simulink model "flyback"  (R2022b)
settings: Solver=FixedStepAuto  StartTime=0.0  StopTime=0.1  FixedStep=1e-7  RelTol=1e-3
values from neighbouring files (symbols this model uses):
  C = Vo*d/(delta_Vc*R*fsw)    (= 0.000104166666667)    [flyback.m]
  d = d*100    (= 37.5)    [flyback.m]
  fsw = 50e3    (= 50000)    [flyback.m]
  Lm = abs(Vin*d/(delta_iL*fsw))    [flyback.m]
  n = 1/5    (= 0.2)    [flyback.m]
  R = Vo^2/Po    (= 7.2)    [flyback.m]
libraries: spsCurrentMeasurementLib x8, spsVoltageMeasurementLib x6, spsParallelRLCBranchLib x3, spsDCVoltageSourceLib x1, spsDiodeLib x1, spsIGBTLib x1, spsVariableRatioTransformerLib x1, sps_lib x1
settings Model: Creator=isild  LastModifiedBy=isild

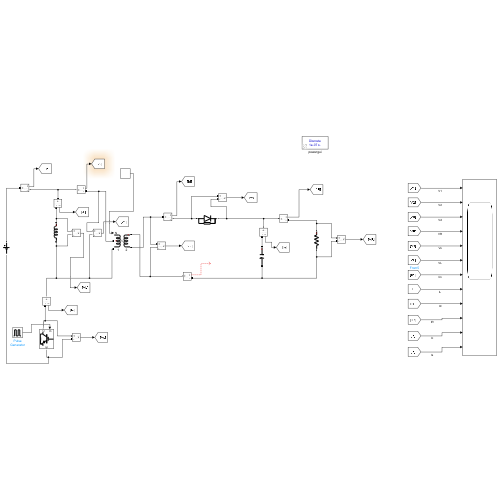
[thumbnail: Simulink's stored preview of the top-level diagram]
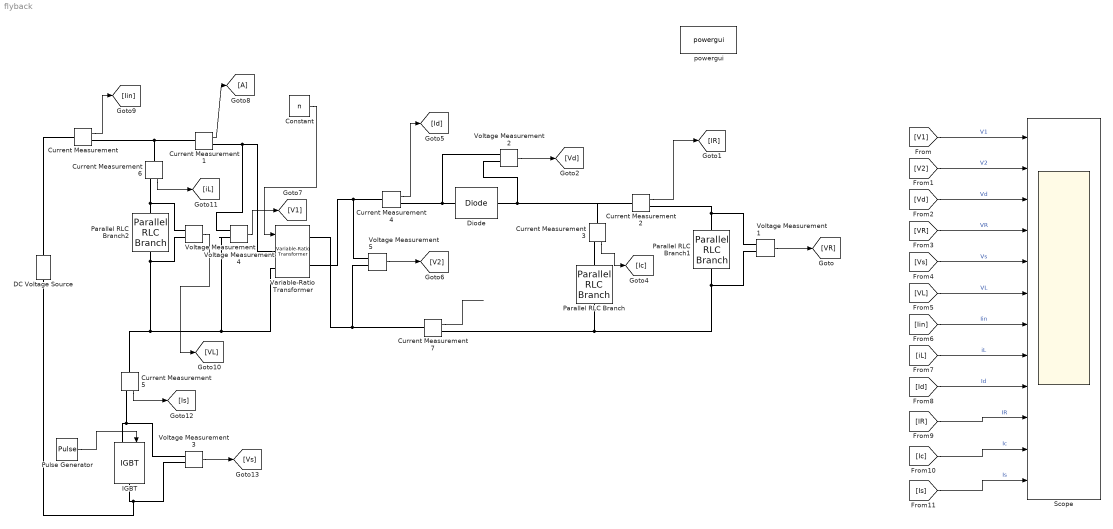
== system flyback ==
  Constant : Constant  Value=n
  Current Measurement{,1..7} (8 alike) : spsCurrentMeasurementLib/Current Measurement  PhasorSimulation=off  OutputType=Complex  PSBequivalent=0
  DC Voltage Source : spsDCVoltageSourceLib/DC Voltage Source  Amplitude=100  Measurements=None
  Diode : spsDiodeLib/Diode  Ron=0.001  Lon=0  Vf=0.8  IC=0  UseSnubber=0  Rs=500  Cs=250e-9  Measurements=off
  Goto8 : Goto
  IGBT : spsIGBTLib/IGBT  Ron=0.001  Lon=0  Vf=1  Tf=1e-6  Tt=2e-6  IC=0  Rs=1e5  Cs=inf  Measurements=off
  Parallel RLC Branch : spsParallelRLCBranchLib/Parallel RLC Branch  LConnTagsString=a  RConnTagsString=__new0  BranchType=C  Resistance=1  Inductance=1e-3  SetiL0=off  InitialCurrent=0  Capacitance=C  Setx0=off  InitialVoltage=0  Measurements=None
  Parallel RLC Branch1 : spsParallelRLCBranchLib/Parallel RLC Branch  LConnTagsString=a  RConnTagsString=__new0  BranchType=R  Resistance=R  Inductance=1e-3  SetiL0=off  InitialCurrent=0  Capacitance=1e-6  Setx0=off  InitialVoltage=0  Measurements=None
  Parallel RLC Branch2 : spsParallelRLCBranchLib/Parallel RLC Branch  LConnTagsString=a  RConnTagsString=__new0  BranchType=L  Resistance=1  Inductance=Lm  SetiL0=off  InitialCurrent=0  Capacitance=1e-6  Setx0=off  InitialVoltage=0  Measurements=None
  Pulse Generator : DiscretePulseGenerator  PulseType=Time based  Period=1/fsw  PulseWidth=d
  Scope : Scope  NumInputPorts=12
  Variable-Ratio Transformer : spsVariableRatioTransformerLib/Variable-Ratio Transformer
      settings: LibrarySourceBlock=|
      | sps_lib/Passives/Variable-Ratio
      | Transformer
  Voltage Measurement{,1..5} (6 alike) : spsVoltageMeasurementLib/Voltage Measurement  PhasorSimulation=off  OutputType=Complex  PSBequivalent=0
  powergui : sps_lib/powergui  Priority=1  SimulationMode=Discrete  SampleTime=1e-7  frequency=60  Iterations=50  frequencyindice=0  Pbase=100e6  ErrMax=1e-4  UnitsV=kV  UnitsW=MW  buscounter=0  FunctionMessages=off  echomessages=off  EnableUseOfTLC=off  CurrentSourceSwitches=off  DisableSnubberDevices=off  DisableRonSwitches=off  DisableVfSwitches=off  DisplayEquations=off  AutomaticDiscreteSolvers=off  SolverType=Tustin/Backward Euler (TBE)  Interpol=off  ExternalGateDelay=off  methode=off  Ts=100  x0status=blocks  SPID=on  SwTol=0  HookPort=off  NonlinearTolerance=1e-4  nMaxIteration=100  ContinueOnMaxIteration=off  RestoreLinks=warning  ResistiveCurrentMeasurement=off  Frange=[0:2:500]  Ylog=off  Xlog=on  ShowGrid=off  save=off  variable=ZData  structure=0  ZoomFFT=off  StartTime=0.0  cycles=1  DisplayStyle=1  fundamental=60  FreqAxis=off  MaxFrequency=1000  frequencyindicesteady=1  RmsSteady=1  display=off
  wires:
  Constant/1 -> Variable-Ratio Transformer/1
  Voltage Measurement1/1 -> [VR]
  Current Measurement2/1 -> [IR]
  Voltage Measurement2/1 -> [Vd]
  Current Measurement7/1 -> ?
  Current Measurement3/1 -> [Ic]
  Current Measurement4/1 -> [Id]
  Voltage Measurement5/1 -> [V2]
  Voltage Measurement4/1 -> [V1]
  Current Measurement1/1 -> Goto8/1
  Current Measurement/1 -> [Iin]
  Voltage Measurement/1 -> [VL]
  Current Measurement6/1 -> [iL]
  Current Measurement5/1 -> [Is]
  Voltage Measurement3/1 -> [Vs]
  [V1] -> Scope/1  "V1"
  [V2] -> Scope/2  "V2"
  [Vd] -> Scope/3  "Vd"
  [VR] -> Scope/4  "VR"
  [Vs] -> Scope/5  "Vs"
  [VL] -> Scope/6  "VL"
  [Iin] -> Scope/7  "Iin"
  [iL] -> Scope/8  "iL"
  [Id] -> Scope/9  "Id"
  [IR] -> Scope/10  "IR"
  [Ic] -> Scope/11  "Ic"
  [Is] -> Scope/12  "Is"
  Pulse Generator/1 -> IGBT/1
  connections:
  Parallel RLC Branch1/LConn1 -- Current Measurement2/RConn1 -- Voltage Measurement1/LConn1
  Parallel RLC Branch1/RConn1 -- Current Measurement7/RConn1 -- Parallel RLC Branch/RConn1 -- Voltage Measurement1/LConn2
  Voltage Measurement2/LConn1 -- Diode/LConn1 -- Current Measurement4/RConn1
  Parallel RLC Branch2/RConn1 -- Voltage Measurement/LConn2 -- Voltage Measurement4/LConn2 -- Variable-Ratio Transformer/LConn2 -- Current Measurement5/LConn1
  Current Measurement/RConn1 -- Current Measurement1/LConn1 -- Current Measurement6/LConn1
  Voltage Measurement3/LConn2 -- IGBT/RConn1 -- DC Voltage Source/LConn1
  DC Voltage Source/RConn1 -- Current Measurement/LConn1
  Current Measurement1/RConn1 -- Voltage Measurement4/LConn1 -- Variable-Ratio Transformer/LConn1
  Voltage Measurement2/LConn2 -- Current Measurement3/LConn1 -- Current Measurement2/LConn1 -- Diode/RConn1
  Current Measurement3/RConn1 -- Parallel RLC Branch/LConn1
  Current Measurement5/RConn1 -- Voltage Measurement3/LConn1 -- IGBT/LConn1
  Parallel RLC Branch2/LConn1 -- Current Measurement6/RConn1 -- Voltage Measurement/LConn1
  Variable-Ratio Transformer/RConn2 -- Voltage Measurement5/LConn1 -- Current Measurement4/LConn1
  Variable-Ratio Transformer/RConn1 -- Voltage Measurement5/LConn2 -- Current Measurement7/LConn1
